simulink model "TST_DYN_ORB"  (R2017b)
settings: Solver=VariableStepAuto  StartTime=0.0  StopTime=10000  RelTol=1e-3
libraries: DYN_GRAV x1, DYN_TRA x1
settings Model: Creator=WilTravis  LastModifiedBy=Mahal

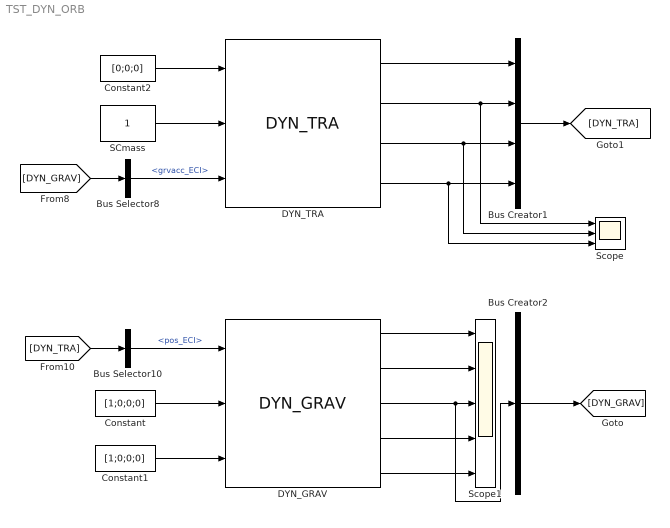
== system TST_DYN_ORB ==
  Bus Creator1 : BusCreator  Inputs=4
  Bus Creator2 : BusCreator  Inputs=1
  Bus Selector10 : BusSelector  OutputSignals=pos_ECI
  Bus Selector8 : BusSelector  OutputSignals=grvacc_ECI
  Constant : Constant  Value=[1;0;0;0]
  Constant1 : Constant  Value=[1;0;0;0]
  Constant2 : Constant  Value=[0;0;0]
  DYN_GRAV : DYN_GRAV/DYN_GRAV
  DYN_TRA : DYN_TRA/DYN_TRA
  SCmass : Constant
  Scope : Scope  NumInputPorts=3
  Scope1 : Scope  NumInputPorts=5
  wires:
  [DYN_GRAV] -> Bus Selector8/1
  Constant2/1 -> DYN_TRA/1
  Bus Selector8/1 -> DYN_TRA/3  "<grvacc_ECI>"
  [DYN_TRA] -> Bus Selector10/1
  DYN_TRA/3 -> Scope/2, Bus Creator1/3
  SCmass/1 -> DYN_TRA/2
  DYN_GRAV/3 -> Bus Creator2/1, Scope1/3
  Bus Selector10/1 -> DYN_GRAV/1  "<pos_ECI>"
  DYN_TRA/2 -> Scope/1, Bus Creator1/2
  DYN_TRA/4 -> Scope/3, Bus Creator1/4
  DYN_TRA/1 -> Bus Creator1/1
  Bus Creator1/1 -> [DYN_TRA]
  Constant/1 -> DYN_GRAV/2
  Constant1/1 -> DYN_GRAV/3
  DYN_GRAV/1 -> Scope1/1
  DYN_GRAV/2 -> Scope1/2
  DYN_GRAV/4 -> Scope1/4
  DYN_GRAV/5 -> Scope1/5
  Bus Creator2/1 -> [DYN_GRAV]
